simulink model "single_phase_vsi_without_pwm_technique"  (R2014a)
settings: Solver=ode23t  StartTime=0.0  StopTime=1  MaxStep=1e-6  RelTol=1e-3
libraries: powerlib x11, powerlib_meascontrol x2
settings Model: Creator=singa  LastModifiedBy=singa

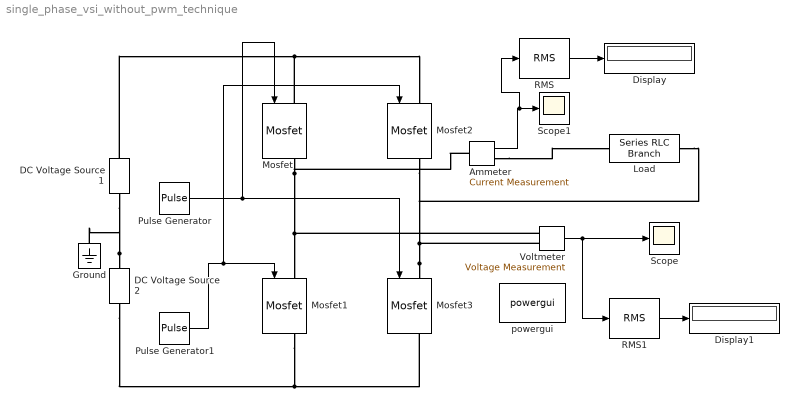
== system single_phase_vsi_without_pwm_technique ==
  Ammeter : powerlib/Measurements/Current Measurement  PhasorSimulation=off  OutputType=Complex  PSBequivalent=0
  DC Voltage Source 1 : powerlib/Electrical Sources/DC Voltage Source  Amplitude=100  Measurements=None
  DC Voltage Source 2 : powerlib/Electrical Sources/DC Voltage Source  Amplitude=100  Measurements=None
  Display : Display
  Display1 : Display
  Ground : powerlib/Elements/Ground  LConnTagsString=a
  Load : powerlib/Elements/Series RLC Branch  LConnTagsString=__new0  RConnTagsString=__new0  BranchType=RL  Resistance=10  Inductance=0.05  SetiL0=off  InitialCurrent=0  Capacitance=1e-6  Setx0=off  InitialVoltage=0  Measurements=None
  Mosfet{,1..3} (4 alike) : powerlib/Power Electronics/Mosfet  Ron=0.1  Lon=0  Rd=0.01  Vfd=0  IC=0  Rs=1e5  Cs=inf  Measurements=on
  Pulse Generator : DiscretePulseGenerator  PulseType=Time based  Period=0.02  PulseWidth=50
  Pulse Generator1 : DiscretePulseGenerator  PulseType=Time based  Period=0.02  PulseWidth=50  PhaseDelay=0.01
  RMS : powerlib_meascontrol/Measurements/RMS  TrueRMS=on  Freq=50  RMSInit=120  Ts=0
  RMS1 : powerlib_meascontrol/Measurements/RMS  TrueRMS=on  Freq=50  RMSInit=120  Ts=0
  Scope : Scope
      settings: YMin=-800  YMax=800  SaveName=line_voltage  SampleInput=on  SampleTime=1e-6
  Scope1 : Scope
      settings: YMin=-800  YMax=800  SaveName=current  SampleInput=on  SampleTime=1e-6
  Voltmeter : powerlib/Measurements/Voltage Measurement  PhasorSimulation=off  OutputType=Complex  PSBequivalent=0
  powergui : powerlib/powergui  Priority=1  SimulationMode=Continuous  SolverType=Tustin  SampleTime=50e-6  frequency=60  SPID=off  DisableSnubberDevices=off  DisableRonSwitches=off  DisableVfSwitches=off  SwTol=0  Interpol=off  DisplayEquations=off  Ts=0  methode=off  frequencyindice=0  Pbase=100e6  ErrMax=1e-4  Iterations=50  UnitsV=kV  UnitsW=MW  FunctionMessages=off  echomessages=off  HookPort=off  EnableUseOfTLC=off  x0status=blocks  RestoreLinks=warning  ResistiveCurrentMeasurement=off  Frange=[0:2:500]  Ylog=off  Xlog=on  ShowGrid=off  save=off  variable=ZData  structure=line_voltage  ZoomFFT=off  StartTime=0.8  cycles=2  DisplayStyle=4  fundamental=50  FreqAxis=on  MaxFrequency=2000  frequencyindicesteady=1  RmsSteady=1  display=off
  wires:
  Voltmeter/1 -> RMS1/1, Scope/1
  Ammeter/1 -> RMS/1, Scope1/1
  Pulse Generator1/1 -> Mosfet2/1, Mosfet1/1
  Pulse Generator/1 -> Mosfet3/1, Mosfet/1
  RMS/1 -> Display/1
  RMS1/1 -> Display1/1
  connections:
  DC Voltage Source 2/RConn1 -- DC Voltage Source 1/LConn1 -- Ground/LConn1
  Ammeter/LConn1 -- Mosfet/RConn1 -- Voltmeter/LConn1 -- Mosfet1/LConn1
  Mosfet3/LConn1 -- Voltmeter/LConn2 -- Mosfet2/RConn1 -- Load/RConn1
  DC Voltage Source 1/RConn1 -- Mosfet/LConn1 -- Mosfet2/LConn1
  DC Voltage Source 2/LConn1 -- Mosfet1/RConn1 -- Mosfet3/RConn1
  Ammeter/RConn1 -- Load/LConn1
